simulink library "IOBlock_Library_TTC580"  (R2021a)
settings: Solver=ode45  StartTime=0.0  StopTime=10.0  RelTol=1e-3
PreLoadFcn:
  | addpath(genpath(fileparts(which('IOBlock_Library_TTC580'))));
  | %addpath(genpath(fileparts(which('IOBlock_Library_TTC580.mdl'))))
  | try
  | addpath(genpath([fileparts(which('IOBlock_Library_TTC580')),'\..\DBC_Importer']));
  | addpath(genpath([fileparts(which('IOBlock_Library_TTC580')),'\..\EEPROM_Importer']));
  | addpath(genpath([fileparts(which('IOBlock_Library_TTC580')),'\..\UserDoc']));
  | catch
  | warning('IOBlock_Library_TTC580: add path to DBC_Importer and EEPROM_Importer manually');
  | end
  | try
  | if exist('..\CustomPackage\scripts\OpenAllPackages.m','file')
  |      run('..\CustomPackage\scripts\OpenAllPackages.m'); %always available, ggf. empty
  | end
  | catch
  | warning('A problem occurred opening automatically the CustomPackage. Please open libraries manually');
  | end
  | try
  | set_param(0,'EditorSmartEditingHotParam','off');
  | catch
  | warning('Simlink preferences for ''Edit key parameter when adding new blocks'' needs to be unchecked manually');
  | end
undefined symbols (not defined in the file or in its folder): ADC_Absolute_10V, ADC_Absolute_32V, ADC_Absolute_5V, ADC_BoardTemp, ADC_ChannelInit, ADC_Current, ADC_Get, ADC_K15_, ADC_Ratiometric_10V, ADC_Ratiometric_5V, ADC_Resistive, ADC_SensorSupply, ADC_UBAT, bit_packing, bit_unpacking, CAN_ConfigMsg, compare2error, compare2FET_PROT_REENABLE, crc32_calc_intern, CRC32_EEPROM_Read, CRC32_EEPROM_Write, DIAG_EnterSafestate, DIAG_Status, DIAG_Status_internal, EEPROM_Mirror, EEPROM_Read, EEPROM_Read_OffsetIn, EEPROM_Read_Raw, EEPROM_Write, EEPROM_Write_OffsetIn, EEPROM_Write_Raw, EnterSafestate, FPU_Handler, Get_DI, Get_DI_VarThreshold, Get_K15_, Get_Pulse_Freq_Curr, Get_Pulse_Freq_Volt, Get_WakeUp, GetDateAndTime, IO_ADC_ResetProtection, IO_Blk_Lib_TTC500, IO_CAN_ReadMsg, IO_CAN_WriteMsg, IO_DI_Get, IO_DI_Init, IO_DI_Init_Var, IO_DO_GetCur, IO_DO_GetVoltage, IO_DO_Init, IO_DO_ResetProtection, IO_DO_Set, IO_Driver_GetSerialNumber, IO_Driver_GetVersionOfDriver, IO_Driver_GetVersionOfFPGA, IO_EEPROM_GetStatus, IO_EEPROM_Init, IO_EEPROM_Read_raw, IO_EEPROM_Write, IO_EEPROM_Write_OffsetIn ... (+73)
libraries: simulink x43
(part 4 of 18)

== system IOBlock_Library_TTC580/PVG and VOUT TTC580 IOlib ==
  Set_PVG_Simple : Subsystem  LoadFcn=|  mask(Set_PVG_Simple_Code){SampleTime=-1, ttlib=IO_Blk_Lib_TTC500, ttDescription=Set_PVG_Simple, tt_iolib_version=0.18, pvg_channel=IO_PVG_00, output_value_init=5000}
      | try
      | %
      | %Upgrade Information - standard BEGIN
      | new_color = 'blue';
      | new_ver = '0.18';
      | act_ver = get_param(gcb,'tt_iolib_version');
      | if not(strcmp(act_ver,new_ver))
      |     disp(['Upgrade block: ',gcb,char(10),'       Version: ',act_ver,' -> ',new_ver]);
      |     %switch - case for specific upgrade information e.g. additional parameter required 
      |     %Change appearance and version information
      |     set_param(gcb,'ForegroundColor',new_color);
      |     set_param(gcb,'tt_iolib_version',new_ver);
      | end
      | %Upgrade Information - standard END
      | catch
      | %Standard catch section BEGIN 
      | disp(' ');
      | disp('------------------------------------------------------------');
      | disp('An error occurred in a callback of the TTC580-BlockLib.');
      | disp(['Please check the parameters in the mask of ',gcb]);
      | disp('If you do not encounter any violations, then please '); 
      | disp('copy the following lines and report this to support@ttcontrol.com ');
      | disp('<< begin of error message dump >>');
      | disp(['Version of TTC580-BlockLib: ', get_param(gcb,'tt_iolib_version')]);
      | disp(get_param(gcb,'ttDescription'));
      | disp(gcb);
      | x=lasterror;disp(x.message);
      | disp(get_param(gcb,'MaskValues'));
      | disp(version);
      | disp(computer);
      | disp('<< end of error message dump >>');
      | disp('------------------------------------------------------------');
      | disp(' ');
      | %Standard catch section END
      | end
      mask help: Sets the output value of one PVG channel in percent * 100
      mask init:
      | %
      settings: CopyFcn=%deleted
      mask Help: web([which('usermanual.html'),'#',lower(get_param(gcb,'ttDescription'))])
      mask TypeOptions pvg_channel: IO_PVG_00 | IO_PVG_01 | IO_PVG_02 | IO_PVG_03 | IO_PVG_04 | IO_PVG_05 | IO_PVG_06 | IO_PVG_07
      mask Callback pvg_channel: %
      mask Callback output_value_init: %
  Set_PVG_VoltFb : Subsystem  LoadFcn=|  mask(Set_PVG_VoltFb_Code){SampleTime=-1, ttlib=IO_Blk_Lib_TTC500, ttDescription=Set_PVG_VoltFb, tt_iolib_version=0.18, pvg_channel=IO_PVG_00, output_value_init=5000}
      | try
      | %
      | %Upgrade Information - standard BEGIN
      | new_color = 'blue';
      | new_ver = '0.18';
      | act_ver = get_param(gcb,'tt_iolib_version');
      | if not(strcmp(act_ver,new_ver))
      |     disp(['Upgrade block: ',gcb,char(10),'       Version: ',act_ver,' -> ',new_ver]);
      |     %switch - case for specific upgrade information e.g. additional parameter required 
      |     %Change appearance and version information
      |     set_param(gcb,'ForegroundColor',new_color);
      |     set_param(gcb,'tt_iolib_version',new_ver);
      | end
      | %Upgrade Information - standard END
      | catch
      | %Standard catch section BEGIN 
      | disp(' ');
      | disp('------------------------------------------------------------');
      | disp('An error occurred in a callback of the TTC580-BlockLib.');
      | disp(['Please check the parameters in the mask of ',gcb]);
      | disp('If you do not encounter any violations, then please '); 
      | disp('copy the following lines and report this to support@ttcontrol.com ');
      | disp('<< begin of error message dump >>');
      | disp(['Version of TTC580-BlockLib: ', get_param(gcb,'tt_iolib_version')]);
      | disp(get_param(gcb,'ttDescription'));
      | disp(gcb);
      | x=lasterror;disp(x.message);
      | disp(get_param(gcb,'MaskValues'));
      | disp(version);
      | disp(computer);
      | disp('<< end of error message dump >>');
      | disp('------------------------------------------------------------');
      | disp(' ');
      | %Standard catch section END
      | end
      mask help:
      | Sets the output value of one PVG channel in percent * 100
      | Output of voltage feedback : 0V..32V
      mask init:
      | %
      settings: CopyFcn=%deleted
      mask Help: web([which('usermanual.html'),'#',lower(get_param(gcb,'ttDescription'))])
      mask TypeOptions pvg_channel: IO_PVG_00 | IO_PVG_01 | IO_PVG_02 | IO_PVG_03 | IO_PVG_04 | IO_PVG_05 | IO_PVG_06 | IO_PVG_07
      mask Callback pvg_channel: %
      mask TypeOptions output_value_init: 1000 | 1100 | 1200 | 1300 | 1400 | 1500 | 1600 | 1700 | 1800 | 1900 | 2000 | 2100 | 2200 | 2300 | 2400 | 2500 | 2600 | 2700 | 2800 | 2900 | 3000 | 3100 | 3200 | 3300 | 3400 | 3500 | 3600 | 3700 | 3800 | 3900 | 4000 | 4100 | 4200 | 4300 | 4400 | 4500 | 4600 | 4700 | 4800 | 4900 | 5000 | 5100 | 5200 | 5300 | 5400 | 5500 | 5600 | 5700 | 5800 | 5900 | 6000 | 6100 | 6200 | 6300 | 6400 | 6500 | 6600 | 6700 | 6800 | 6900 | 7000 | 7100 | 7200 | 7300 | 7400 | 7500 | 7600 | 7700 | 7800 | 7900 | 8000 | 8100 | 8200 | 8300 | 8400 | 8500 | 8600 | 8700 | 8800 | 8900 | 9000
      mask Callback output_value_init: %
  Set_VOUT_Simple : Subsystem  LoadFcn=|  mask(Set_VOUT_Simple_Code){SampleTime=-1, ttlib=IO_Blk_Lib_TTC500, ttDescription=Set_VOUT_Simple, tt_iolib_version=0.18, vout_channel=IO_VOUT_00}
      | try
      | %
      | %Upgrade Information - standard BEGIN
      | new_color = 'blue';
      | new_ver = '0.18';
      | act_ver = get_param(gcb,'tt_iolib_version');
      | if not(strcmp(act_ver,new_ver))
      |     disp(['Upgrade block: ',gcb,char(10),'       Version: ',act_ver,' -> ',new_ver]);
      |     %switch - case for specific upgrade information e.g. additional parameter required 
      |     %Change appearance and version information
      |     set_param(gcb,'ForegroundColor',new_color);
      |     set_param(gcb,'tt_iolib_version',new_ver);
      | end
      | %Upgrade Information - standard END
      | catch
      | %Standard catch section BEGIN 
      | disp(' ');
      | disp('------------------------------------------------------------');
      | disp('An error occurred in a callback of the TTC580-BlockLib.');
      | disp(['Please check the parameters in the mask of ',gcb]);
      | disp('If you do not encounter any violations, then please '); 
      | disp('copy the following lines and report this to support@ttcontrol.com ');
      | disp('<< begin of error message dump >>');
      | disp(['Version of TTC580-BlockLib: ', get_param(gcb,'tt_iolib_version')]);
      | disp(get_param(gcb,'ttDescription'));
      | disp(gcb);
      | x=lasterror;disp(x.message);
      | disp(get_param(gcb,'MaskValues'));
      | disp(version);
      | disp(computer);
      | disp('<< end of error message dump >>');
      | disp('------------------------------------------------------------');
      | disp(' ');
      | %Standard catch section END
      | end
      mask help: Sets the output voltage of one voltage output channel. 0..32V
      mask init:
      | %
      settings: CopyFcn=%deleted
      mask Help: web([which('usermanual.html'),'#',lower(get_param(gcb,'ttDescription'))])
      mask TypeOptions vout_channel: IO_VOUT_00 | IO_VOUT_01 | IO_VOUT_02 | IO_VOUT_03 | IO_VOUT_04 | IO_VOUT_05 | IO_VOUT_06 | IO_VOUT_07
      mask Callback vout_channel: %
  Set_VOUT_VoltFb : Subsystem  LoadFcn=|  mask(Set_VOUT_VoltFb_Code){SampleTime=-1, ttlib=IO_Blk_Lib_TTC500, ttDescription=Set_VOUT_VoltFb, tt_iolib_version=0.18, vout_channel=IO_VOUT_00}
      | try
      | %
      | %Upgrade Information - standard BEGIN
      | new_color = 'blue';
      | new_ver = '0.18';
      | act_ver = get_param(gcb,'tt_iolib_version');
      | if not(strcmp(act_ver,new_ver))
      |     disp(['Upgrade block: ',gcb,char(10),'       Version: ',act_ver,' -> ',new_ver]);
      |     %switch - case for specific upgrade information e.g. additional parameter required 
      |     %Change appearance and version information
      |     set_param(gcb,'ForegroundColor',new_color);
      |     set_param(gcb,'tt_iolib_version',new_ver);
      | end
      | %Upgrade Information - standard END
      | catch
      | %Standard catch section BEGIN 
      | disp(' ');
      | disp('------------------------------------------------------------');
      | disp('An error occurred in a callback of the TTC580-BlockLib.');
      | disp(['Please check the parameters in the mask of ',gcb]);
      | disp('If you do not encounter any violations, then please '); 
      | disp('copy the following lines and report this to support@ttcontrol.com ');
      | disp('<< begin of error message dump >>');
      | disp(['Version of TTC580-BlockLib: ', get_param(gcb,'tt_iolib_version')]);
      | disp(get_param(gcb,'ttDescription'));
      | disp(gcb);
      | x=lasterror;disp(x.message);
      | disp(get_param(gcb,'MaskValues'));
      | disp(version);
      | disp(computer);
      | disp('<< end of error message dump >>');
      | disp('------------------------------------------------------------');
      | disp(' ');
      | %Standard catch section END
      | end
      mask help:
      | Sets the output voltage of one voltage output channel in mV (range [0..32000])
      | returning the measured voltage in mV (range: 0..32000)
      mask init:
      | %
      settings: CopyFcn=%deleted
      mask Help: web([which('usermanual.html'),'#',lower(get_param(gcb,'ttDescription'))])
      mask TypeOptions vout_channel: IO_VOUT_00 | IO_VOUT_01 | IO_VOUT_02 | IO_VOUT_03 | IO_VOUT_04 | IO_VOUT_05 | IO_VOUT_06 | IO_VOUT_07
      mask Callback vout_channel: %

== system IOBlock_Library_TTC580/PWD Blocks TTC580 IOlib ==
  Get_Pulse_Freq_Curr : Subsystem  LoadFcn=|  mask(Get_Pulse_Freq_Curr_Code){SampleTime=-1, ttlib=IO_Blk_Lib_TTC500, ttDescription=Get_Pulse_Freq_Curr, tt_iolib_version=0.26, timer_channel=IO_PWD_00, pulse_mode=IO_PWD_HIGH_TIME, freq_mode=IO_PWD_RISING_VAR, capture_count=1, pupd=IO_PWD_PD_90}
      | try
      | %
      | %Upgrade Information - standard BEGIN
      | new_color = 'blue';
      | new_ver = '0.26';
      | act_ver = get_param(gcb,'tt_iolib_version');
      | if not(strcmp(act_ver,new_ver))
      |     disp(['Upgrade block: ',gcb,char(10),'       Version: ',act_ver,' to ',new_ver]);
      |     %switch - case for specific upgrade information e.g. additional parameter required 
      |     %Change appearance and version information
      |     set_param(gcb,'ForegroundColor',new_color);
      |     set_param(gcb,'tt_iolib_version',new_ver);
      | end
      | %Upgrade Information - standard END
      | catch
      | %Standard catch section BEGIN
      | errordlg('An error occurred in a callback of the TTC580-BlockLib. Please open the Diagnostic Viewer for further details');
      | disp(' ');
      | disp('------------------------------------------------------------');
      | disp('An error occurred in a callback of the TTC580-BlockLib.');
      | disp(['Please check the parameters in the mask of ',gcb]);
      | disp('If you do not encounter any violations, then please '); 
      | disp('copy the following lines and report this to support@ttcontrol.com ');
      | disp('<< begin of error message dump >>');
      | disp(['Version of TTC580-BlockLib: ', get_param(gcb,'tt_iolib_version')]);
      | disp(get_param(gcb,'ttDescription'));
      | disp(gcb);
      | x=lasterror;disp(x.message);
      | disp(get_param(gcb,'MaskValues'));
      | disp(version);
      | disp(computer);
      | disp('<< end of error message dump >>');
      | disp('------------------------------------------------------------');
      | disp(' ');
      | %Standard catch section END
      | end
      mask help: Get the frequency and the pulse-width from the specified timer channel connected to a current sensor (7mA/14mA)
      mask init: same as IOBlock_Library_TTC580/ADC Blocks TTC580 IOlib/ADC_Absolute_10V
      settings: CopyFcn=%deleted
      mask Help: web([which('usermanual.html'),'#',lower(get_param(gcb,'ttDescription'))])
      mask TypeOptions timer_channel: IO_PWD_00 | IO_PWD_01 | IO_PWD_02 | IO_PWD_03 | IO_PWD_04 | IO_PWD_05
      mask Callback timer_channel: %
      mask TypeOptions pulse_mode: IO_PWD_HIGH_TIME | IO_PWD_LOW_TIME | IO_PWD_PERIOD_TIME
      mask Callback pulse_mode: %
      mask TypeOptions freq_mode: IO_PWD_RISING_VAR | IO_PWD_FALLING_VAR
      mask Callback freq_mode: %
      mask Callback capture_count: %
      mask Callback pupd: %
  Get_Pulse_Freq_Volt : Subsystem  LoadFcn=|  mask(Get_Pulse_Freq_Volt_Code){SampleTime=-1, ttlib=IO_Blk_Lib_TTC500, ttDescription=Get_Pulse_Freq_Volt, tt_iolib_version=0.26, timer_channel=IO_PWD_00, pulse_mode=IO_PWD_HIGH_TIME, freq_mode=IO_PWD_RISING_VAR, capture_count=1, pupd=IO_PWD_PU_10K}
      | try
      | %
      | %Upgrade Information - standard BEGIN
      | new_color = 'blue';
      | new_ver = '0.26';
      | act_ver = get_param(gcb,'tt_iolib_version');
      | if not(strcmp(act_ver,new_ver))
      |     disp(['Upgrade block: ',gcb,char(10),'       Version: ',act_ver,' to ',new_ver]);
      |     %switch - case for specific upgrade information e.g. additional parameter required 
      |     %Change appearance and version information
      |     set_param(gcb,'ForegroundColor',new_color);
      |     set_param(gcb,'tt_iolib_version',new_ver);
      | end
      | %Upgrade Information - standard END
      | catch
      | %Standard catch section BEGIN
      | errordlg('An error occurred in a callback of the TTC580-BlockLib. Please open the Diagnostic Viewer for further details');
      | disp(' ');
      | disp('------------------------------------------------------------');
      | disp('An error occurred in a callback of the TTC580-BlockLib.');
      | disp(['Please check the parameters in the mask of ',gcb]);
      | disp('If you do not encounter any violations, then please '); 
      | disp('copy the following lines and report this to support@ttcontrol.com ');
      | disp('<< begin of error message dump >>');
      | disp(['Version of TTC580-BlockLib: ', get_param(gcb,'tt_iolib_version')]);
      | disp(get_param(gcb,'ttDescription'));
      | disp(gcb);
      | x=lasterror;disp(x.message);
      | disp(get_param(gcb,'MaskValues'));
      | disp(version);
      | disp(computer);
      | disp('<< end of error message dump >>');
      | disp('------------------------------------------------------------');
      | disp(' ');
      | %Standard catch section END
      | end
      mask help: Get the frequency and the pulse-width from the specified timer channel driven by a voltage signal.
      mask init: same as IOBlock_Library_TTC580/ADC Blocks TTC580 IOlib/ADC_Absolute_10V
      settings: CopyFcn=%deleted
      mask Help: web([which('usermanual.html'),'#',lower(get_param(gcb,'ttDescription'))])
      mask TypeOptions timer_channel: IO_PWD_00 | IO_PWD_01 | IO_PWD_02 | IO_PWD_03 | IO_PWD_04 | IO_PWD_05 | IO_PWD_06 | IO_PWD_07 | IO_PWD_08 | IO_PWD_09 | IO_PWD_10 | IO_PWD_11 | IO_PWD_12 | IO_PWD_13 | IO_PWD_14 | IO_PWD_15 | IO_PWD_16 | IO_PWD_17 | IO_PWD_18 | IO_PWD_19
      mask Callback timer_channel:
      | try
      | s_ParameterDecision = 'timer_channel'; %Deside on this parameter
      | cc_ValuesDecision={{'IO_PWD_12','IO_PWD_13','IO_PWD_14','IO_PWD_15','IO_PWD_16','IO_PWD_17','IO_PWD_18','IO_PWD_19'}}; %Positive DescitionValues
      | s_ParameterGrey = 'pupd'; %Gray out this
      | c_ValueGrey = {'IO_PWD_PU_10K'};   %Fixed value
      | %trim
      | s_ParameterDecision = strtrim(s_ParameterDecision);
      | cc_ValuesDecision = strtrim(cc_ValuesDecision);
      | s_ParameterGrey = strtrim(s_ParameterGrey);
      | c_ValueGrey = strtrim(c_ValueGrey);
      | c_MaskEnables=get_param(gcb,'MaskEnables');
      | %check consistency
      | if length(cc_ValuesDecision)~= length(c_ValueGrey),disp('DevCode: 012');end
      | idx=strmatch(s_ParameterGrey,get_param(gcb,'MaskNames'));
      | c_MaskEnables{idx}='on'; %default
      |     for i = 1: length(cc_ValuesDecision)
      |         if ~isempty(strmatch(get_param(gcb, s_ParameterDecision), cc_ValuesDecision{i},'exact'))
      |            set_param(gcb, s_ParameterGrey, c_ValueGrey{i});
      |            c_MaskEnables{idx}='off';
      |         end
      |     end
      | set_param(gcb,'MaskEnables',c_MaskEnables);
      | catch
      | %Standard catch section BEGIN
      | errordlg('An error occurred in a callback of the TTC580-BlockLib. Please open the Diagnostic Viewer for further details');
      | disp(' ');
      | disp('------------------------------------------------------------');
      | disp('An error occurred in a callback of the TTC580-BlockLib.');
      | disp(['Please check the parameters in the mask of ',gcb]);
      | disp('If you do not encounter any violations, then please ');
      | disp('copy the following lines and report this to support@ttcontrol.com ');
      | disp('<< begin of error message dump >>');
      | disp(['Version of TTC580-BlockLib: ', get_param(gcb,'tt_iolib_version')]);
      | disp(get_param(gcb,'ttDescription'));
      | disp(gcb);
      | x=lasterror;disp(x.message);
      | disp(get_param(gcb,'MaskValues'));
      | disp(version);
      | disp(computer);
      | disp('<< end of error message dump >>');
      | disp('------------------------------------------------------------');
      | disp(' ');
      | %Standard catch section END
      | end
      mask TypeOptions pulse_mode: IO_PWD_HIGH_TIME | IO_PWD_LOW_TIME | IO_PWD_PERIOD_TIME
      mask Callback pulse_mode: %
      mask TypeOptions freq_mode: IO_PWD_RISING_VAR | IO_PWD_FALLING_VAR
      mask Callback freq_mode: %
      mask Callback capture_count: %
      mask TypeOptions pupd: IO_PWD_PU_10K | IO_PWD_PD_10K
      mask Callback pupd: %
  PWD_Inc : Subsystem  LoadFcn=|  mask(PWD_Inc_Code){SampleTime=-1, ttlib=IO_Blk_Lib_TTC500, ttDescription=PWD_Inc, tt_iolib_version=0.26, inc_channel=IO_PWD_00, secondary_channel=IO_PWD_01, mode=IO_PWD_INC_2_COUNT, pupd=IO_PWD_PU_10K}
      | try
      | %
      | %Upgrade Information - standard BEGIN
      | new_color = 'blue';
      | new_ver = '0.26';
      | act_ver = get_param(gcb,'tt_iolib_version');
      | if not(strcmp(act_ver,new_ver))
      |     disp(['Upgrade block: ',gcb,char(10),'       Version: ',act_ver,' to ',new_ver]);
      |     %switch - case for specific upgrade information e.g. additional parameter required 
      |     %Change appearance and version information
      |     set_param(gcb,'ForegroundColor',new_color);
      |     set_param(gcb,'tt_iolib_version',new_ver);
      | end
      | %Upgrade Information - standard END
      | catch
      | %Standard catch section BEGIN
      | errordlg('An error occurred in a callback of the TTC580-BlockLib. Please open the Diagnostic Viewer for further details');
      | disp(' ');
      | disp('------------------------------------------------------------');
      | disp('An error occurred in a callback of the TTC580-BlockLib.');
      | disp(['Please check the parameters in the mask of ',gcb]);
      | disp('If you do not encounter any violations, then please '); 
      | disp('copy the following lines and report this to support@ttcontrol.com ');
      | disp('<< begin of error message dump >>');
      | disp(['Version of TTC580-BlockLib: ', get_param(gcb,'tt_iolib_version')]);
      | disp(get_param(gcb,'ttDescription'));
      | disp(gcb);
      | x=lasterror;disp(x.message);
      | disp(get_param(gcb,'MaskValues'));
      | disp(version);
      | disp(computer);
      | disp('<< end of error message dump >>');
      | disp('------------------------------------------------------------');
      | disp(' ');
      | %Standard catch section END
      | end
      mask help: Setup a single incremental interface and get the counter value. Two PWD channels are needed for one incremental interface
      mask init: same as IOBlock_Library_TTC580/ADC Blocks TTC580 IOlib/ADC_Absolute_10V
      settings: CopyFcn=%deleted
      mask Help: web([which('usermanual.html'),'#',lower(get_param(gcb,'ttDescription'))])
      mask TypeOptions inc_channel: IO_PWD_00 | IO_PWD_02 | IO_PWD_04 | IO_PWD_06 | IO_PWD_08 | IO_PWD_10
      mask Callback inc_channel:
      | try
      | s_ParameterDecision = 'inc_channel'; %Deside on this parameter
      | cc_ValuesDecision={{'IO_PWD_00'},{'IO_PWD_02'},{'IO_PWD_04'},{'IO_PWD_06'},{'IO_PWD_08'},{'IO_PWD_10'}}; %Positive DescitionValues
      | s_ParameterGrey = 'secondary_channel'; %Gray out this
      | c_ValueGrey = {'IO_PWD_01','IO_PWD_03','IO_PWD_05','IO_PWD_07','IO_PWD_09','IO_PWD_11'};   %Fixed value
      | %trim
      | s_ParameterDecision = strtrim(s_ParameterDecision);
      | cc_ValuesDecision = strtrim(cc_ValuesDecision);
      | s_ParameterGrey = strtrim(s_ParameterGrey);
      | c_ValueGrey = strtrim(c_ValueGrey);
      | c_MaskEnables=get_param(gcb,'MaskEnables');
      | %check consistency
      | if length(cc_ValuesDecision)~= length(c_ValueGrey),disp('DevCode: 012');end
      | idx=strmatch(s_ParameterGrey,get_param(gcb,'MaskNames'));
      | c_MaskEnables{idx}='on'; %default
      |     for i = 1: length(cc_ValuesDecision)
      |         if ~isempty(strmatch(get_param(gcb, s_ParameterDecision), cc_ValuesDecision{i},'exact'))
      |            set_param(gcb, s_ParameterGrey, c_ValueGrey{i});
      |            c_MaskEnables{idx}='off';
      |         end
      |     end
      | set_param(gcb,'MaskEnables',c_MaskEnables);
      | catch
      | %Standard catch section BEGIN
      | errordlg('An error occurred in a callback of the TTC580-BlockLib. Please open the Diagnostic Viewer for further details');
      | disp(' ');
      | disp('------------------------------------------------------------');
      | disp('An error occurred in a callback of the TTC580-BlockLib.');
      | disp(['Please check the parameters in the mask of ',gcb]);
      | disp('If you do not encounter any violations, then please ');
      | disp('copy the following lines and report this to support@ttcontrol.com ');
      | disp('<< begin of error message dump >>');
      | disp(['Version of TTC580-BlockLib: ', get_param(gcb,'tt_iolib_version')]);
      | disp(get_param(gcb,'ttDescription'));
      | disp(gcb);
      | x=lasterror;disp(x.message);
      | disp(get_param(gcb,'MaskValues'));
      | disp(version);
      | disp(computer);
      | disp('<< end of error message dump >>');
      | disp('------------------------------------------------------------');
      | disp(' ');
      | %Standard catch section END
      | end
      mask Callback secondary_channel: %
      mask TypeOptions mode: IO_PWD_INC_1_COUNT | IO_PWD_INC_2_COUNT
      mask Callback mode: %
      mask TypeOptions pupd: IO_PWD_PU_10K | IO_PWD_PD_10K
      mask Callback pupd: %
  PWD_IncReset : Subsystem  LoadFcn=|  mask(PWD_IncReset_Code){SampleTime=-1, ttlib=IO_Blk_Lib_TTC500, ttDescription=PWD_IncReset, tt_iolib_version=0.26, inc_channel=IO_PWD_00, count=0}
      | try
      | %
      | %Upgrade Information - standard BEGIN
      | new_color = 'blue';
      | new_ver = '0.26';
      | act_ver = get_param(gcb,'tt_iolib_version');
      | if not(strcmp(act_ver,new_ver))
      |     disp(['Upgrade block: ',gcb,char(10),'       Version: ',act_ver,' to ',new_ver]);
      |     %switch - case for specific upgrade information e.g. additional parameter required 
      |     %Change appearance and version information
      |     set_param(gcb,'ForegroundColor',new_color);
      |     set_param(gcb,'tt_iolib_version',new_ver);
      | end
      | %Upgrade Information - standard END
      | catch
      | %Standard catch section BEGIN
      | errordlg('An error occurred in a callback of the TTC580-BlockLib. Please open the Diagnostic Viewer for further details');
      | disp(' ');
      | disp('------------------------------------------------------------');
      | disp('An error occurred in a callback of the TTC580-BlockLib.');
      | disp(['Please check the parameters in the mask of ',gcb]);
      | disp('If you do not encounter any violations, then please '); 
      | disp('copy the following lines and report this to support@ttcontrol.com ');
      | disp('<< begin of error message dump >>');
      | disp(['Version of TTC580-BlockLib: ', get_param(gcb,'tt_iolib_version')]);
      | disp(get_param(gcb,'ttDescription'));
      | disp(gcb);
      | x=lasterror;disp(x.message);
      | disp(get_param(gcb,'MaskValues'));
      | disp(version);
      | disp(computer);
      | disp('<< end of error message dump >>');
      | disp('------------------------------------------------------------');
      | disp(' ');
      | %Standard catch section END
      | end
      mask help: Set the counter value of an incremental interface to the value given by the parameter "count"
      mask init: same as IOBlock_Library_TTC580/ADC Blocks TTC580 IOlib/ADC_Absolute_10V
      settings: CopyFcn=%deleted
      mask Help: web([which('usermanual.html'),'#',lower(get_param(gcb,'ttDescription'))])
      mask TypeOptions inc_channel: IO_PWD_00 | IO_PWD_02 | IO_PWD_04 | IO_PWD_06 | IO_PWD_08 | IO_PWD_10
      mask Callback inc_channel: %
      mask Callback count: %

== system IOBlock_Library_TTC580/PWM Blocks TTC580 IOlib ==
  Set_PWM_CurrFb : Subsystem  LoadFcn=|  mask(Set_PWM_CurrFb_Code){SampleTime=-1, ttlib=IO_Blk_Lib_TTC500, ttDescription=Set_PWM_CurrFb, tt_iolib_version=0.26, pwm_channel=IO_PWM_00, frequency=100, polarity_high=TRUE, diag_margin=on}
      | try
      | %
      | %Upgrade Information - standard BEGIN
      | new_color = 'blue';
      | new_ver = '0.26';
      | act_ver = get_param(gcb,'tt_iolib_version');
      | if not(strcmp(act_ver,new_ver))
      |     disp(['Upgrade block: ',gcb,char(10),'       Version: ',act_ver,' to ',new_ver]);
      |     %switch - case for specific upgrade information e.g. additional parameter required 
      |     %Change appearance and version information
      |     set_param(gcb,'ForegroundColor',new_color);
      |     set_param(gcb,'tt_iolib_version',new_ver);
      | end
      | %Upgrade Information - standard END
      | catch
      | %Standard catch section BEGIN
      | errordlg('An error occurred in a callback of the TTC580-BlockLib. Please open the Diagnostic Viewer for further details');
      | disp(' ');
      | disp('------------------------------------------------------------');
      | disp('An error occurred in a callback of the TTC580-BlockLib.');
      | disp(['Please check the parameters in the mask of ',gcb]);
      | disp('If you do not encounter any violations, then please '); 
      | disp('copy the following lines and report this to support@ttcontrol.com ');
      | disp('<< begin of error message dump >>');
      | disp(['Version of TTC580-BlockLib: ', get_param(gcb,'tt_iolib_version')]);
      | disp(get_param(gcb,'ttDescription'));
      | disp(gcb);
      | x=lasterror;disp(x.message);
      | disp(get_param(gcb,'MaskValues'));
      | disp(version);
      | disp(computer);
      | disp('<< end of error message dump >>');
      | disp('------------------------------------------------------------');
      | disp(' ');
      | %Standard catch section END
      | end
      mask help: Set the duty cycle for a PWM channel (range [0..65535]) with the high output signal set variable and returning the measured current in mA (range [0A .. 7.5A] )
      mask init: same as IOBlock_Library_TTC580/ADC Blocks TTC580 IOlib/ADC_Absolute_10V
      settings: CopyFcn=%deleted
      mask Help: web([which('usermanual.html'),'#',lower(get_param(gcb,'ttDescription'))])
      mask TypeOptions pwm_channel: IO_PWM_00 | IO_PWM_01 | IO_PWM_02 | IO_PWM_03 | IO_PWM_04 | IO_PWM_05 | IO_PWM_06 | IO_PWM_07 | IO_PWM_08 | IO_PWM_09 | IO_PWM_10 | IO_PWM_11 | IO_PWM_12 | IO_PWM_13 | IO_PWM_14 | IO_PWM_15 | IO_PWM_16 | IO_PWM_17 | IO_PWM_18 | IO_PWM_19 | IO_PWM_20 | IO_PWM_21 | IO_PWM_22 | IO_PWM_23 | IO_PWM_24 | IO_PWM_25 | IO_PWM_26 | IO_PWM_27 | IO_PWM_28 | IO_PWM_29 | IO_PWM_30 | IO_PWM_31 | IO_PWM_32 | IO_PWM_33 | IO_PWM_34 | IO_PWM_35
      mask Callback pwm_channel: %
      mask TypeOptions frequency: 1000 | 800 | 666 | 571 | 500 | 444 | 400 | 363 | 333 | 307 | 285 | 266 | 250 | 235 | 222 | 210 | 200 | 181 | 166 | 153 | 142 | 133 | 125 | 117 | 111 | 105 | 100 | 90 | 83 | 76 | 71 | 66 | 62 | 58 | 55 | 52 | 50
      mask Callback frequency: %
      mask Callback polarity_high: %
      mask Callback diag_margin: %
  Set_PWM_FullFb : Subsystem  LoadFcn=|  mask(Set_PWM_FullFb_Code){SampleTime=-1, ttlib=IO_Blk_Lib_TTC500, ttDescription=Set_PWM_FullFb, tt_iolib_version=0.26, pwm_channel=IO_PWM_00, frequency=100, polarity_high=on, diag_margin=on}
      | try
      | %
      | %Upgrade Information - standard BEGIN
      | new_color = 'blue';
      | new_ver = '0.26';
      | act_ver = get_param(gcb,'tt_iolib_version');
      | if not(strcmp(act_ver,new_ver))
      |     disp(['Upgrade block: ',gcb,char(10),'       Version: ',act_ver,' to ',new_ver]);
      |     %switch - case for specific upgrade information e.g. additional parameter required 
      |     %Change appearance and version information
      |     set_param(gcb,'ForegroundColor',new_color);
      |     set_param(gcb,'tt_iolib_version',new_ver);
      | end
      | %Upgrade Information - standard END
      | catch
      | %Standard catch section BEGIN
      | errordlg('An error occurred in a callback of the TTC580-BlockLib. Please open the Diagnostic Viewer for further details');
      | disp(' ');
      | disp('------------------------------------------------------------');
      | disp('An error occurred in a callback of the TTC580-BlockLib.');
      | disp(['Please check the parameters in the mask of ',gcb]);
      | disp('If you do not encounter any violations, then please '); 
      | disp('copy the following lines and report this to support@ttcontrol.com ');
      | disp('<< begin of error message dump >>');
      | disp(['Version of TTC580-BlockLib: ', get_param(gcb,'tt_iolib_version')]);
      | disp(get_param(gcb,'ttDescription'));
      | disp(gcb);
      | x=lasterror;disp(x.message);
      | disp(get_param(gcb,'MaskValues'));
      | disp(version);
      | disp(computer);
      | disp('<< end of error message dump >>');
      | disp('------------------------------------------------------------');
      | disp(' ');
      | %Standard catch section END
      | end
      mask help:
      | Set the duty cycle for a PWM channel (range [0..65535]) , returning:
      | 1) Measured current in mA (Range: 0..7500 (=0A .. 7.500A) )
      | 2) High time feedback in us
      | 3) Period feedback in us
      mask init: same as IOBlock_Library_TTC580/ADC Blocks TTC580 IOlib/ADC_Absolute_10V
      settings: CopyFcn=%deleted
      mask Help: web([which('usermanual.html'),'#',lower(get_param(gcb,'ttDescription'))])
      mask TypeOptions pwm_channel: IO_PWM_00 | IO_PWM_01 | IO_PWM_02 | IO_PWM_03 | IO_PWM_04 | IO_PWM_05 | IO_PWM_06 | IO_PWM_07 | IO_PWM_08 | IO_PWM_09 | IO_PWM_10 | IO_PWM_11 | IO_PWM_12 | IO_PWM_13 | IO_PWM_14 | IO_PWM_15 | IO_PWM_16 | IO_PWM_17 | IO_PWM_18 | IO_PWM_19 | IO_PWM_20 | IO_PWM_21 | IO_PWM_22 | IO_PWM_23 | IO_PWM_24 | IO_PWM_25 | IO_PWM_26 | IO_PWM_27 | IO_PWM_28 | IO_PWM_29 | IO_PWM_30 | IO_PWM_31 | IO_PWM_32 | IO_PWM_33 | IO_PWM_34 | IO_PWM_35
      mask Callback pwm_channel: %
      mask TypeOptions frequency: 1000 | 800 | 666 | 571 | 500 | 444 | 400 | 363 | 333 | 307 | 285 | 266 | 250 | 235 | 222 | 210 | 200 | 181 | 166 | 153 | 142 | 133 | 125 | 117 | 111 | 105 | 100 | 90 | 83 | 76 | 71 | 66 | 62 | 58 | 55 | 52 | 50
      mask Callback frequency: %
      mask Callback polarity_high: %
      mask Callback diag_margin: %
  Set_PWM_Simple : Subsystem  LoadFcn=|  mask(Set_PWM_Simple_Code){SampleTime=-1, ttlib=IO_Blk_Lib_TTC500, ttDescription=Set_PWM_Simple, tt_iolib_version=0.26, pwm_channel=IO_PWM_00, frequency=100, polarity_high=TRUE, diag_margin=FALSE}
      | try
      | %specific upgrade to 0.12
      | if (0.12 > str2num(get_param(gcb,'tt_iolib_version'))) || (0.8 == str2num(get_param(gcb,'tt_iolib_version')))
      |    set_param(gcb,'diag_margin','FALSE'); 
      | end
      | %Upgrade Information - standard BEGIN
      | new_color = 'blue';
      | new_ver = '0.26';
      | act_ver = get_param(gcb,'tt_iolib_version');
      | if not(strcmp(act_ver,new_ver))
      |     disp(['Upgrade block: ',gcb,char(10),'       Version: ',act_ver,' to ',new_ver]);
      |     %switch - case for specific upgrade information e.g. additional parameter required 
      |     %Change appearance and version information
      |     set_param(gcb,'ForegroundColor',new_color);
      |     set_param(gcb,'tt_iolib_version',new_ver);
      | end
      | %Upgrade Information - standard END
      | catch
      | %Standard catch section BEGIN
      | errordlg('An error occurred in a callback of the TTC580-BlockLib. Please open the Diagnostic Viewer for further details');
      | disp(' ');
      | disp('------------------------------------------------------------');
      | disp('An error occurred in a callback of the TTC580-BlockLib.');
      | disp(['Please check the parameters in the mask of ',gcb]);
      | disp('If you do not encounter any violations, then please '); 
      | disp('copy the following lines and report this to support@ttcontrol.com ');
      | disp('<< begin of error message dump >>');
      | disp(['Version of TTC580-BlockLib: ', get_param(gcb,'tt_iolib_version')]);
      | disp(get_param(gcb,'ttDescription'));
      | disp(gcb);
      | x=lasterror;disp(x.message);
      | disp(get_param(gcb,'MaskValues'));
      | disp(version);
      | disp(computer);
      | disp('<< end of error message dump >>');
      | disp('------------------------------------------------------------');
      | disp(' ');
      | %Standard catch section END
      | end
      mask help: Set the duty cycle for a PWM channel within the range [0..65535] (=0..100%)
      mask init: same as IOBlock_Library_TTC580/ADC Blocks TTC580 IOlib/ADC_Absolute_10V
      settings: CopyFcn=%deleted
      mask Help: web([which('usermanual.html'),'#',lower(get_param(gcb,'ttDescription'))])
      mask TypeOptions pwm_channel: IO_PWM_00 | IO_PWM_01 | IO_PWM_02 | IO_PWM_03 | IO_PWM_04 | IO_PWM_05 | IO_PWM_06 | IO_PWM_07 | IO_PWM_08 | IO_PWM_09 | IO_PWM_10 | IO_PWM_11 | IO_PWM_12 | IO_PWM_13 | IO_PWM_14 | IO_PWM_15 | IO_PWM_16 | IO_PWM_17 | IO_PWM_18 | IO_PWM_19 | IO_PWM_20 | IO_PWM_21 | IO_PWM_22 | IO_PWM_23 | IO_PWM_24 | IO_PWM_25 | IO_PWM_26 | IO_PWM_27 | IO_PWM_28 | IO_PWM_29 | IO_PWM_30 | IO_PWM_31 | IO_PWM_32 | IO_PWM_33 | IO_PWM_34 | IO_PWM_35
      mask Callback pwm_channel: %
      mask TypeOptions frequency: 1000 | 800 | 666 | 571 | 500 | 444 | 400 | 363 | 333 | 307 | 285 | 266 | 250 | 235 | 222 | 210 | 200 | 181 | 166 | 153 | 142 | 133 | 125 | 117 | 111 | 105 | 100 | 90 | 83 | 76 | 71 | 66 | 62 | 58 | 55 | 52 | 50
      mask Callback frequency: %
      mask Callback polarity_high: %
      mask Callback diag_margin: %

== system IOBlock_Library_TTC580/SensorSupply TTC580 IOlib ==
  SensorSupply_5V : Subsystem  LoadFcn=|  mask(SensorSupply_5V_Code){SampleTime=-1, ttlib=IO_Blk_Lib_TTC500, ttDescription=SensorSupply_5V, tt_iolib_version=0.26, sensor_supply=IO_SENSOR_SUPPLY_0}
      | try
      | %specific upgrade to 0.17
      | if (0.17 > str2num(get_param(gcb,'tt_iolib_version'))) || (0.8 == str2num(get_param(gcb,'tt_iolib_version')))
      |     warning('off','Simulink:SL_RefBlockUnknownParameter');   %R2007b: no parameter.mode available in mask any more
      |     warning('off','Simulink:blocks:RefBlockUnknownParameter'); %same for R2014
      | end
      | %Upgrade Information - standard BEGIN
      | new_color = 'blue';
      | new_ver = '0.26';
      | act_ver = get_param(gcb,'tt_iolib_version');
      | if not(strcmp(act_ver,new_ver))
      |     disp(['Upgrade block: ',gcb,char(10),'       Version: ',act_ver,' to ',new_ver]);
      |     %switch - case for specific upgrade information e.g. additional parameter required 
      |     %Change appearance and version information
      |     set_param(gcb,'ForegroundColor',new_color);
      |     set_param(gcb,'tt_iolib_version',new_ver);
      | end
      | %Upgrade Information - standard END
      | catch
      | %Standard catch section BEGIN
      | errordlg('An error occurred in a callback of the TTC580-BlockLib. Please open the Diagnostic Viewer for further details');
      | disp(' ');
      | disp('------------------------------------------------------------');
      | disp('An error occurred in a callback of the TTC580-BlockLib.');
      | disp(['Please check the parameters in the mask of ',gcb]);
      | disp('If you do not encounter any violations, then please '); 
      | disp('copy the following lines and report this to support@ttcontrol.com ');
      | disp('<< begin of error message dump >>');
      | disp(['Version of TTC580-BlockLib: ', get_param(gcb,'tt_iolib_version')]);
      | disp(get_param(gcb,'ttDescription'));
      | disp(gcb);
      | x=lasterror;disp(x.message);
      | disp(get_param(gcb,'MaskValues'));
      | disp(version);
      | disp(computer);
      | disp('<< end of error message dump >>');
      | disp('------------------------------------------------------------');
      | disp(' ');
      | %Standard catch section END
      | end
      mask help: Switch on sensor supply 0 or sensor supply 1 with fixed 5 volts
      mask init: same as IOBlock_Library_TTC580/ADC Blocks TTC580 IOlib/ADC_Absolute_10V
      settings: CopyFcn=%deleted
      mask Help: web([which('usermanual.html'),'#',lower(get_param(gcb,'ttDescription'))])
      mask TypeOptions sensor_supply: IO_SENSOR_SUPPLY_0 | IO_SENSOR_SUPPLY_1
      mask Callback sensor_supply: %
  SensorSupply_Modif : Subsystem  LoadFcn=|  mask(SensorSupply_Modif_Code){SampleTime=-1, ttlib=IO_Blk_Lib_TTC500, ttDescription=SensorSupply_Modif, tt_iolib_version=0.26, sensor_supply=IO_SENSOR_SUPPLY_2}
      | try
      | %
      | %Upgrade Information - standard BEGIN
      | new_color = 'blue';
      | new_ver = '0.26';
      | act_ver = get_param(gcb,'tt_iolib_version');
      | if not(strcmp(act_ver,new_ver))
      |     disp(['Upgrade block: ',gcb,char(10),'       Version: ',act_ver,' to ',new_ver]);
      |     %switch - case for specific upgrade information e.g. additional parameter required 
      |     %Change appearance and version information
      |     set_param(gcb,'ForegroundColor',new_color);
      |     set_param(gcb,'tt_iolib_version',new_ver);
      | end
      | %Upgrade Information - standard END
      | catch
      | %Standard catch section BEGIN
      | errordlg('An error occurred in a callback of the TTC580-BlockLib. Please open the Diagnostic Viewer for further details');
      | disp(' ');
      | disp('------------------------------------------------------------');
      | disp('An error occurred in a callback of the TTC580-BlockLib.');
      | disp(['Please check the parameters in the mask of ',gcb]);
      | disp('If you do not encounter any violations, then please '); 
      | disp('copy the following lines and report this to support@ttcontrol.com ');
      | disp('<< begin of error message dump >>');
      | disp(['Version of TTC580-BlockLib: ', get_param(gcb,'tt_iolib_version')]);
      | disp(get_param(gcb,'ttDescription'));
      | disp(gcb);
      | x=lasterror;disp(x.message);
      | disp(get_param(gcb,'MaskValues'));
      | disp(version);
      | disp(computer);
      | disp('<< end of error message dump >>');
      | disp('------------------------------------------------------------');
      | disp(' ');
      | %Standard catch section END
      | end
      mask help: Operate sensor supply 2 configurable by the input with the possible values [0,5,6,7,8,9,10] volts
      mask init:
      | %
      settings: CopyFcn=%deleted
      mask Help: web([which('usermanual.html'),'#',lower(get_param(gcb,'ttDescription'))])
      mask Callback sensor_supply: %
